simulink model "simulation_basic_working"  (R2022b)
settings: Solver=ode4  StartTime=0.0  StopTime=30  FixedStep=5e-7  MaxStep=1e-6  RelTol=1e-3
undefined symbols (not defined in the file or in its folder): control, inverter, motor, speed
libraries: mcbcontrolslib x5, slpidlib x3, SignalEditorBlockLib x2, spsTriangleGeneratorLib x1
settings Model: Creator=Rizwan Sadik  LastModifiedBy=Rizwan Sadik

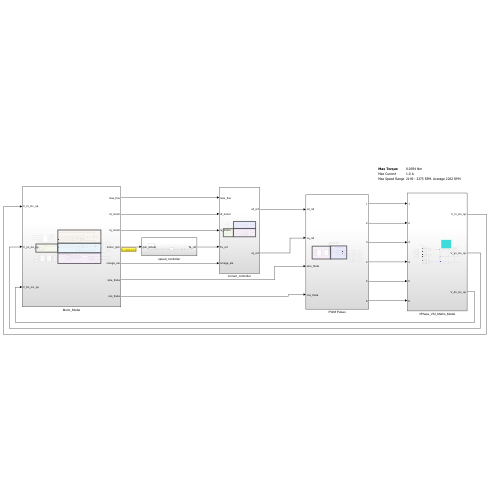
[thumbnail: Simulink's stored preview of the top-level diagram]
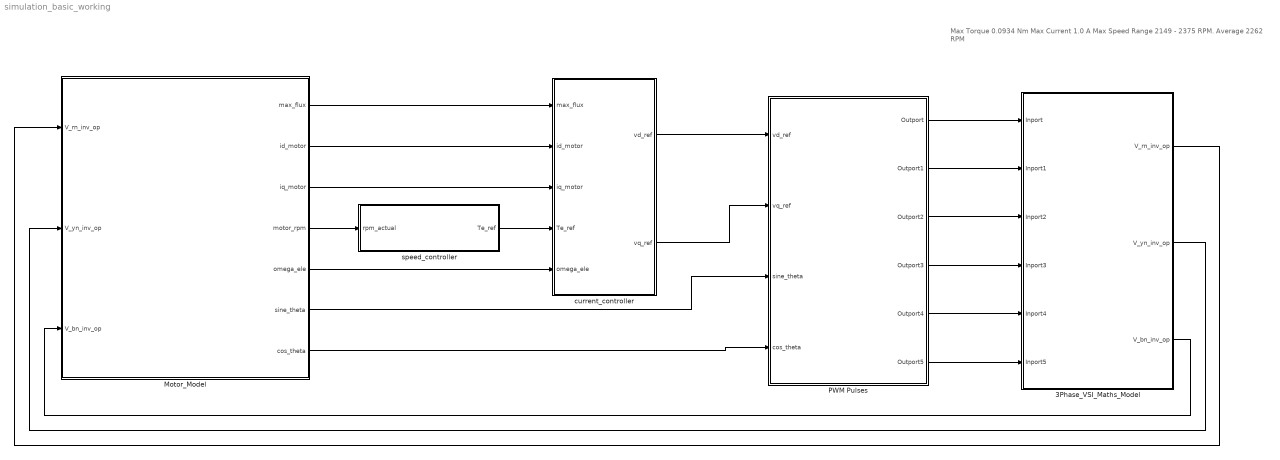
== system simulation_basic_working ==
  note: Max Torque
      | 0.0934 Nm
      |
      | Max Current
      | 1.0 A
      |
      | Max Speed Range
      | 2149 - 2375 RPM. Average 2262 RPM
  3Phase_VSI_Maths_Model : Subsystem  Description=|
      | Input DC Voltage = Vdc
      | Ouput Phase Voltages = Vrn, Vyn, Vbn
      | 
      | Pole Voltage = Vdc/2
      | Pole Voltages - instantaneous values:
      | Vro = +- Vdc/2
      | Vyo = +- Vdc/2
      | Vbo = +- Vdc/2
      | 
      | Leg 1 o/p is Vr. Switches 1 & 4
      | sw 1 ON (sw 4 OFF) -> Vro = +Vdc/2
      | sw 4 ON (sw 1 OFF) -> Vro = -Vdc/2
      | 
      | Leg 2 o/p is Vy. Switches 3 & 6
      | sw 3 ON (sw 6 OFF) -> Vyo = +Vdc/2
      | sw 6 ON (sw 3 OFF) -> Vyo = -Vdc/2
      | 
      | Leg 3 o/p is Vb. Switches 5 & 2
      | sw 5 ON (sw 2 OFF) -> Vbo = +Vdc/2
      | sw 2 ON (sw 5 OFF) -> Vbo = -Vdc/2
      | 
      | Vrn = (2Vro-Vyo-Vbo)/3
      | Vyn = (2Vyo-Vro-Vbo)/3
      | Vbn =(2Vbo-Vyo-Vro)/3
  Motor_Model : Subsystem
  PWM Pulses : Subsystem
  current_controller : Subsystem
  speed_controller : Subsystem
  wires:
  speed_controller/1(Te_ref) -> current_controller/4(Te_ref)
  Motor_Model/5(omega_ele) -> current_controller/5(omega_ele)
  PWM Pulses/1(Outport) -> 3Phase_VSI_Maths_Model/1(Inport)
  Motor_Model/1(max_flux) -> current_controller/1(max_flux)
  PWM Pulses/4(Outport3) -> 3Phase_VSI_Maths_Model/4(Inport3)
  PWM Pulses/5(Outport4) -> 3Phase_VSI_Maths_Model/5(Inport4)
  Motor_Model/6(sine_theta) -> PWM Pulses/3(sine_theta)
  PWM Pulses/3(Outport2) -> 3Phase_VSI_Maths_Model/3(Inport2)
  Motor_Model/3(iq_motor) -> current_controller/3(iq_motor)
  PWM Pulses/2(Outport1) -> 3Phase_VSI_Maths_Model/2(Inport1)
  PWM Pulses/6(Outport5) -> 3Phase_VSI_Maths_Model/6(Inport5)
  Motor_Model/2(id_motor) -> current_controller/2(id_motor)
  Motor_Model/7(cos_theta) -> PWM Pulses/4(cos_theta)
  current_controller/2(vq_ref) -> PWM Pulses/2(vq_ref)
  current_controller/1(vd_ref) -> PWM Pulses/1(vd_ref)
  3Phase_VSI_Maths_Model/3(V_bn_inv_op) -> Motor_Model/3(V_bn_inv_op)
  3Phase_VSI_Maths_Model/2(V_yn_inv_op) -> Motor_Model/2(V_yn_inv_op)
  3Phase_VSI_Maths_Model/1(V_rn_inv_op) -> Motor_Model/1(V_rn_inv_op)
  Motor_Model/4(motor_rpm) -> speed_controller/1(rpm_actual)

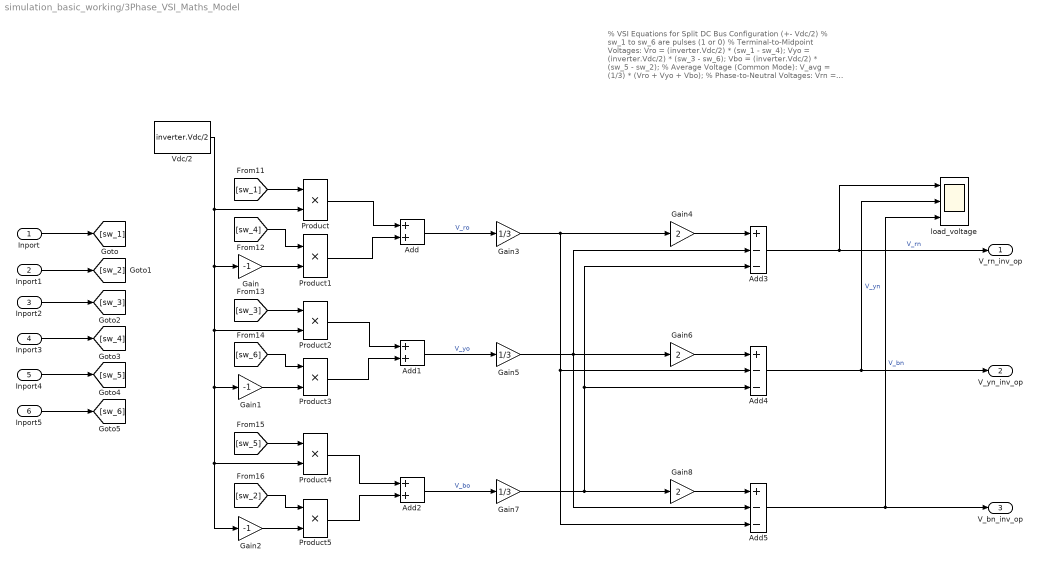
== system simulation_basic_working/3Phase_VSI_Maths_Model ==
  note: % VSI Equations for Split DC Bus Configuration (+- Vdc/2)
      | % sw_1 to sw_6 are pulses (1 or 0)
      |
      | % Terminal-to-Midpoint Voltages:
      | Vro = (inverter.Vdc/2) * (sw_1 - sw_4);
      | Vyo = (inverter.Vdc/2) * (sw_3 - sw_6);
      | Vbo = (inverter.Vdc/2) * (sw_5 - sw_2);
      |
      | % Average Voltage (Common Mode):
      | V_avg = (1/3) * (Vro + Vyo + Vbo);
      |
      | % Phase-to-Neutral Voltages:
      | Vrn = Vro - V_avg;
      | Vyn = Vyo - V_avg;
      | Vbn = Vbo - V_avg;
  Inport : Inport
  Inport1 : Inport  Port=2
  Inport2 : Inport  Port=3
  Inport3 : Inport  Port=4
  Inport4 : Inport  Port=5
  Inport5 : Inport  Port=6
  Add : Sum
  Add1 : Sum
  Add2 : Sum
  Add3 : Sum  Inputs=+--
  Add4 : Sum  Inputs=+--
  Add5 : Sum  Inputs=+--
  Gain : Gain  Gain=-1
  Gain1 : Gain  Gain=-1
  Gain2 : Gain  Gain=-1
  Gain3 : Gain  Gain=1/3
  Gain4 : Gain  Gain=2
  Gain5 : Gain  Gain=1/3
  Gain6 : Gain  Gain=2
  Gain7 : Gain  Gain=1/3
  Gain8 : Gain  Gain=2
  Product{,1..5} (6 alike) : Product
  Vdc/2 : Constant  Value=inverter.Vdc/2
  load_voltage : Scope  NumInputPorts=3
  V_rn_inv_op : Outport
  V_yn_inv_op : Outport  Port=2
  V_bn_inv_op : Outport  Port=3
  wires:
  Product2/1 -> Add1/1
  Add3/1 -> load_voltage/1, V_rn_inv_op/1  "V_rn"
  Product/1 -> Add/1
  Product4/1 -> Add2/1
  Vdc/2/1 -> Gain2/1, Product4/2, Gain1/1, Product2/2, Gain/1, Product/2
  Gain3/1 -> Add5/3, Add4/2, Gain4/1
  Add4/1 -> load_voltage/2, V_yn_inv_op/1  "V_yn"
  [sw_5] -> Product4/1
  Add/1 -> Gain3/1  "V_ro"
  Gain8/1 -> Add5/1
  Add2/1 -> Gain7/1  "V_bo"
  Gain7/1 -> Gain8/1, Add3/3, Add4/3
  Product5/1 -> Add2/2
  Gain5/1 -> Add5/2, Gain6/1, Add3/2
  [sw_3] -> Product2/1
  Gain4/1 -> Add3/1
  [sw_6] -> Product3/1
  Product3/1 -> Add1/2
  [sw_2] -> Product5/1
  Gain1/1 -> Product3/2
  Gain/1 -> Product1/2
  Product1/1 -> Add/2
  [sw_4] -> Product1/1
  [sw_1] -> Product/1
  Gain2/1 -> Product5/2
  Gain6/1 -> Add4/1
  Add5/1 -> V_bn_inv_op/1, load_voltage/3  "V_bn"
  Inport/1 -> [sw_1]
  Inport1/1 -> [sw_2]
  Inport3/1 -> [sw_4]
  Inport2/1 -> [sw_3]
  Inport5/1 -> [sw_6]
  Inport4/1 -> [sw_5]
  Add1/1 -> Gain5/1  "V_yo"

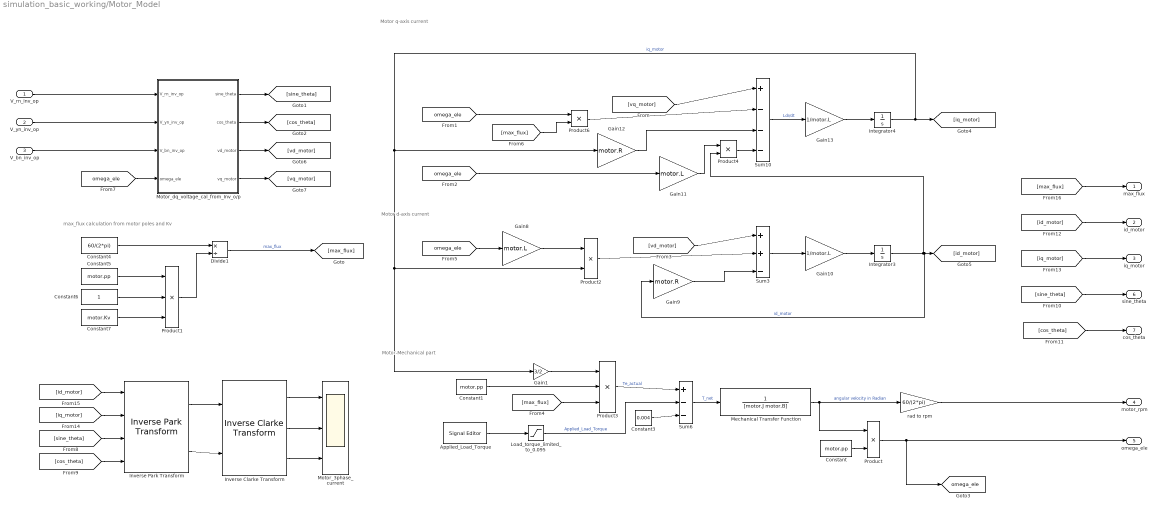
== system simulation_basic_working/Motor_Model ==
  note: max_flux calculation from motor poles and Kv
  note: Motor-Mechanical part
  note: Motor d-axis current
  note: Motor q-axis current
  V_rn_inv_op : Inport
  V_yn_inv_op : Inport  Port=2
  V_bn_inv_op : Inport  Port=3
  Applied_Load_Torque : SignalEditorBlockLib/Signal Editor  FileName=signal_editor.mat  ActiveScenario=Scenario  ActiveSignal=1  IsBus=off  OutputBusObjectStr=Bus: BusObject  SampleTime=0  ZeroCross=off  OutputAfterFinalValue=Setting to zero  Unit=inherit  PreserveSignalName=on
  Constant : Constant  Value=motor.pp
  Constant1 : Constant  Value=motor.pp
  Constant3 : Constant  Value=0.004
  Constant4 : Constant  Value=60/(2*pi)
  Constant5 : Constant  Value=motor.pp
  Constant6 : Constant
  Constant7 : Constant  Value=motor.Kv
  Divide1 : Product  Inputs=*/
  Gain1 : Gain  Gain=3/2
  Gain10 : Gain  Gain=1/motor.L
  Gain11 : Gain  Gain=motor.L
  Gain12 : Gain  Gain=motor.R
  Gain13 : Gain  Gain=1/motor.L
  Gain8 : Gain  Gain=motor.L
  Gain9 : Gain  Gain=motor.R
  Integrator3 : Integrator
  Integrator4 : Integrator
  Inverse Clarke Transform : mcbcontrolslib/Inverse Clarke Transform
      settings: LibrarySourceBlock=mcbhdllib/Controls/Math Transforms/Inverse Clarke Transform
  Inverse Park Transform : mcbcontrolslib/Inverse Park Transform  AxisAlignment=D-axis
      settings: LibrarySourceBlock=mcblib/Controls/Math Transforms/Inverse Park Transform
  Load_torque_limited_to_0.095 : Saturate  UpperLimit=0.095  LowerLimit=0
  Mechanical Transfer Function : TransferFcn  Denominator=[motor.J motor.B]
  Motor_3phase_current : Scope  NumInputPorts=3
  Motor_dq_voltage_cal_from_Inv_o/p : Subsystem
  Product{,2,4,6} (4 alike) : Product
  Product1 : Product  Inputs=3
  Product3 : Product  Inputs=3
  Sum10 : Sum  Inputs=|+---
  Sum3 : Sum  Inputs=|++-
  Sum6 : Sum  Inputs=+|--
  rad to rpm : Gain  Gain=60/(2*pi)
  max_flux : Outport
  id_motor : Outport  Port=2
  iq_motor : Outport  Port=3
  motor_rpm : Outport  Port=4
  omega_ele : Outport  Port=5
  sine_theta : Outport  Port=6
  cos_theta : Outport  Port=7
  tag scope: omega_ele=global
  wires:
  Product6/1 -> Sum10/2
  Gain12/1 -> Sum10/3
  [max_flux] -> Product6/2
  Gain13/1 -> Integrator4/1
  Gain11/1 -> Product4/1
  Integrator4/1 -> [iq_motor], Gain1/1, Product2/2, Gain12/1  "iq_motor"
  Product4/1 -> Sum10/4
  [omega_ele] -> Gain11/1
  Sum10/1 -> Gain13/1  "Ldi/dt​​"
  [vq_motor] -> Sum10/1
  [omega_ele] -> Product6/1
  Product2/1 -> Sum3/2
  Integrator3/1 -> [id_motor], Gain9/1, Product4/2  "id_motor"
  Gain9/1 -> Sum3/3
  Gain8/1 -> Product2/1
  Sum3/1 -> Gain10/1
  Gain10/1 -> Integrator3/1
  [omega_ele] -> Gain8/1
  [vd_motor] -> Sum3/1
  [max_flux] -> Product3/3
  Constant/1 -> Product/2
  Product/1 -> omega_ele/1, [omega_ele]
  Mechanical Transfer Function/1 -> rad to rpm/1, Product/1  "angular velocity in Radian"
  Sum6/1 -> Mechanical Transfer Function/1  "T_net"
  Constant3/1 -> Sum6/3
  Gain1/1 -> Product3/1
  Product3/1 -> Sum6/1  "Te_actual"
  Load_torque_limited_to_0.095/1 -> Sum6/2  "Applied_Load_Torque"
  Constant1/1 -> Product3/2
  rad to rpm/1 -> motor_rpm/1
  Constant6/1 -> Product1/2
  Product1/1 -> Divide1/2
  Constant5/1 -> Product1/1
  Constant7/1 -> Product1/3
  Constant4/1 -> Divide1/1
  Divide1/1 -> [max_flux]  "max_flux"
  Applied_Load_Torque/1 -> Load_torque_limited_to_0.095/1
  V_rn_inv_op/1 -> Motor_dq_voltage_cal_from_Inv_o/p/1(V_rn_inv_op)
  V_yn_inv_op/1 -> Motor_dq_voltage_cal_from_Inv_o/p/2(V_yn_inv_op)
  V_bn_inv_op/1 -> Motor_dq_voltage_cal_from_Inv_o/p/3(V_bn_inv_op)
  [omega_ele] -> Motor_dq_voltage_cal_from_Inv_o/p/4(omega_ele)
  Motor_dq_voltage_cal_from_Inv_o/p/2(cos_theta) -> [cos_theta]
  Motor_dq_voltage_cal_from_Inv_o/p/3(vd_motor) -> [vd_motor]
  Motor_dq_voltage_cal_from_Inv_o/p/4(vq_motor) -> [vq_motor]
  Inverse Clarke Transform/2 -> Motor_3phase_current/2
  Inverse Clarke Transform/1 -> Motor_3phase_current/1
  Inverse Park Transform/1 -> Inverse Clarke Transform/1
  Inverse Clarke Transform/3 -> Motor_3phase_current/3
  Inverse Park Transform/2 -> Inverse Clarke Transform/2
  Motor_dq_voltage_cal_from_Inv_o/p/1(sine_theta) -> [sine_theta]
  [sine_theta] -> Inverse Park Transform/3
  [cos_theta] -> Inverse Park Transform/4
  [sine_theta] -> sine_theta/1
  [cos_theta] -> cos_theta/1
  [id_motor] -> id_motor/1
  [iq_motor] -> iq_motor/1
  [iq_motor] -> Inverse Park Transform/2
  [id_motor] -> Inverse Park Transform/1
  [max_flux] -> max_flux/1

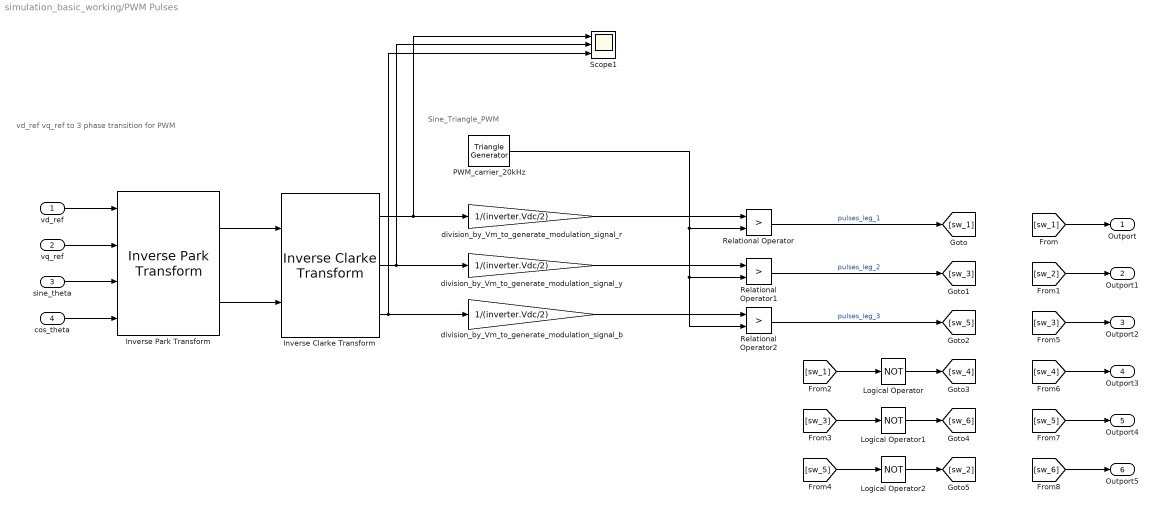
== system simulation_basic_working/PWM Pulses ==
  note: vd_ref vq_ref to 3 phase transition for PWM
  note: Sine_Triangle_PWM
  vd_ref : Inport
  vq_ref : Inport  Port=2
  sine_theta : Inport  Port=3
  cos_theta : Inport  Port=4
  Inverse Clarke Transform : mcbcontrolslib/Inverse Clarke Transform
      settings: LibrarySourceBlock=mcbhdllib/Controls/Math Transforms/Inverse Clarke Transform
  Inverse Park Transform : mcbcontrolslib/Inverse Park Transform  AxisAlignment=D-axis
      settings: LibrarySourceBlock=mcblib/Controls/Math Transforms/Inverse Park Transform
  Logical Operator : Logic  Operator=NOT  AllPortsSameDT=off  OutDataTypeStr=boolean
  Logical Operator1 : Logic  Operator=NOT  AllPortsSameDT=off  OutDataTypeStr=boolean
  Logical Operator2 : Logic  Operator=NOT  AllPortsSameDT=off  OutDataTypeStr=boolean
  PWM_carrier_20kHz : spsTriangleGeneratorLib/Triangle Generator  Freq=20000  Phase=0  Ts=0
  Relational Operator : RelationalOperator  Operator=>  OutDataTypeStr=boolean  RndMeth=Simplest  InputSameDT=off
  Relational Operator1 : RelationalOperator  Operator=>  OutDataTypeStr=boolean  RndMeth=Simplest  InputSameDT=off
  Relational Operator2 : RelationalOperator  Operator=>  OutDataTypeStr=boolean  RndMeth=Simplest  InputSameDT=off
  Scope1 : Scope  NumInputPorts=3
  division_by_Vm_to_generate_modulation_signal_b : Gain  Gain=1/(inverter.Vdc/2)
  division_by_Vm_to_generate_modulation_signal_r : Gain  Gain=1/(inverter.Vdc/2)
  division_by_Vm_to_generate_modulation_signal_y : Gain  Gain=1/(inverter.Vdc/2)
  Outport : Outport
  Outport1 : Outport  Port=2
  Outport2 : Outport  Port=3
  Outport3 : Outport  Port=4
  Outport4 : Outport  Port=5
  Outport5 : Outport  Port=6
  wires:
  [sw_3] -> Logical Operator1/1
  Logical Operator2/1 -> [sw_2]
  cos_theta/1 -> Inverse Park Transform/4
  sine_theta/1 -> Inverse Park Transform/3
  [sw_5] -> Logical Operator2/1
  Inverse Park Transform/2 -> Inverse Clarke Transform/2
  Inverse Park Transform/1 -> Inverse Clarke Transform/1
  Logical Operator/1 -> [sw_4]
  Logical Operator1/1 -> [sw_6]
  [sw_1] -> Logical Operator/1
  vd_ref/1 -> Inverse Park Transform/1
  vq_ref/1 -> Inverse Park Transform/2
  [sw_1] -> Outport/1
  [sw_6] -> Outport5/1
  [sw_2] -> Outport1/1
  [sw_3] -> Outport2/1
  [sw_4] -> Outport3/1
  [sw_5] -> Outport4/1
  Relational Operator2/1 -> [sw_5]  "pulses_leg_3"
  Relational Operator1/1 -> [sw_3]  "pulses_leg_2"
  Relational Operator/1 -> [sw_1]  "pulses_leg_1"
  PWM_carrier_20kHz/1 -> Relational Operator2/2, Relational Operator1/2, Relational Operator/2
  division_by_Vm_to_generate_modulation_signal_y/1 -> Relational Operator1/1
  division_by_Vm_to_generate_modulation_signal_b/1 -> Relational Operator2/1
  Inverse Clarke Transform/3 -> Scope1/3, division_by_Vm_to_generate_modulation_signal_b/1
  Inverse Clarke Transform/2 -> Scope1/2, division_by_Vm_to_generate_modulation_signal_y/1
  division_by_Vm_to_generate_modulation_signal_r/1 -> Relational Operator/1
  Inverse Clarke Transform/1 -> Scope1/1, division_by_Vm_to_generate_modulation_signal_r/1

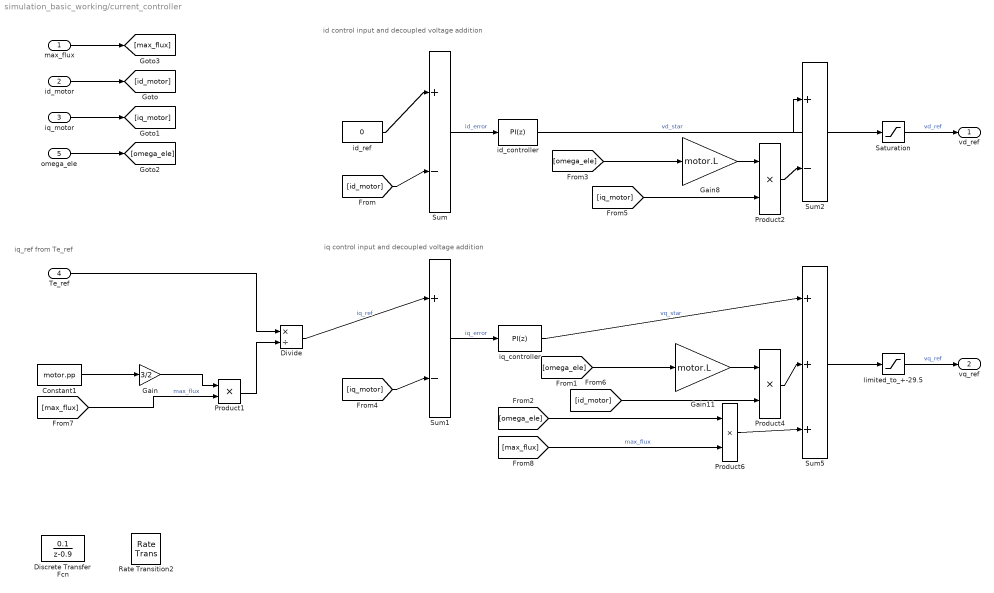
== system simulation_basic_working/current_controller ==
  note: iq_ref from Te_ref
  note: iq control input and decoupled voltage addition
  note: id control input and decoupled voltage addition
  max_flux : Inport
  id_motor : Inport  Port=2
  iq_motor : Inport  Port=3
  Te_ref : Inport  Port=4  SampleTime=5e-4
  omega_ele : Inport  Port=5
  Constant1 : Constant  Value=motor.pp
  Discrete Transfer Fcn : DiscreteTransferFcn  Numerator=[0.1]  Denominator=[1 -0.9]  SampleTime=5e-5
  Divide : Product  Inputs=*/
  Gain : Gain  Gain=3/2
  Gain11 : Gain  Gain=motor.L
  Gain8 : Gain  Gain=motor.L
  Product{1..2,4,6} (4 alike) : Product
  Rate Transition2 : RateTransition  Integrity=off  OutPortSampleTime=5e-5
  Saturation : Saturate  UpperLimit=29.5  LowerLimit=-29.5
  Sum : Sum  Inputs=|+-
  Sum1 : Sum  Inputs=|+-
  Sum2 : Sum  Inputs=|+-
  Sum5 : Sum  Inputs=|+++
  id_controller : slpidlib/PID Controller  Controller=PI  Form=Parallel  TimeDomain=Discrete-time  UseExternalTs=off  SampleTime=5e-5  IntegratorMethod=Forward Euler  FilterMethod=Forward Euler  ControllerParametersSource=internal  P=control.Kp  I=control.Ki  UseKiTs=off  D=0  N=100  UseFilter=on  TunerSelectOption=Transfer Function Based (PID Tuner App)  InitialConditionSource=internal  InitialConditionForIntegrator=0  InitialConditionForFilter=0  DifferentiatorICPrevScaledInput=0  ExternalReset=none  TrackingMode=off  Kt=1  LimitOutput=on  SatLimitsSource=internal  UpperSaturationLimit=inf  LowerSaturationLimit=-inf  LinearizeAsGain=on  AntiWindupMode=clamping  Kb=1  LimitIntegrator=off  UpperIntegratorSaturationLimit=inf  LowerIntegratorSaturationLimit=-inf  POutMin=[]  POutMax=[]  IOutMin=[]  IOutMax=[]  DOutMin=[]  DOutMax=[]  NOutMin=[]  NOutMax=[]  SumOutMin=[]  SumOutMax=[]  SaturationOutMin=[]  SaturationOutMax=[]  PParamMin=[]  PParamMax=[]  IParamMin=[]  IParamMax=[]  DParamMin=[]  DParamMax=[]  NParamMin=[]  NParamMax=[]  KbParamMin=[]  KbParamMax=[]  KtParamMin=[]  KtParamMax=[]  KbOutMin=[]  KbOutMax=[]  KtOutMin=[]  KtOutMax=[]  IntegratorOutMin=[]  IntegratorOutMax=[]  FilterOutMin=[]  FilterOutMax=[]  SumI1OutMin=[]  SumI1OutMax=[]  SumI2OutMin=[]  SumI2OutMax=[]  SumI3OutMin=[]  SumI3OutMax=[]  SumI4OutMin=[]  SumI4OutMax=[]  SumDOutMin=[]  SumDOutMax=[]  DifferentiatorOutMin=[]  DifferentiatorOutMax=[]  FilterDiffOutCoefMin=[]  FilterDiffOutCoefMax=[]  ReciprocalOutMin=[]  ReciprocalOutMax=[]  SumDenOutMin=[]  SumDenOutMax=[]  SumNumOutMin=[]  SumNumOutMax=[]  DivideOutMin=[]  DivideOutMax=[]  UdiffTsProdOutMin=[]  UdiffTsProdOutMax=[]  NTsProdOutMin=[]  NTsProdOutMax=[]  UintegralTsProdOutMin=[]  UintegralTsProdOutMax=[]  UngainTsProdOutMin=[]  UngainTsProdOutMax=[]  ClampingZeroOutDataTypeStr=Inherit: Inherit via back propagation  ClampingZeroOutMin=[]  ClampingZeroOutMax=[]  FilterDenConstantOutDataTypeStr=Inherit: Inherit via back propagation  FilterDenConstantOutMin=[]  FilterDenConstantOutMax=[]  PCopyOutDataTypeStr=Inherit: Inherit via back propagation  PCopyOutMin=[]  PCopyOutMax=[]  NCopyOutDataTypeStr=Inherit: Inherit via back propagation  NCopyOutMin=[]  NCopyOutMax=[]  IntegratorContinuousStateAttributes=''  IntegratorStateMustResolveToSignalObject=off  IntegratorRTWStateStorageClass=Auto  FilterContinuousStateAttributes=''  FilterStateMustResolveToSignalObject=off  FilterRTWStateStorageClass=Auto  ParallelPVariant=InternalParameters  IdealPVariant=Disabled  IVariant=InternalParameters  DVariant=Disabled  IntegratorVariant=Discrete  SatVariant=Enabled  AWVariant=DiscClampingParallel  PCopyVariant=Disabled  TRVariant=Disabled  FdbkBlocksVariant=Forward  IdealPFdbkVariant=Disabled  SatFdbkVariant=Disabled  DerivativeFilterVariant=Disabled  NVariant=Disabled  NCopyVariant=Disabled_SignalSpec  FilterICVariant=Disabled  IntegratorICVariant=InternalICs  ExternalResetVariant=Disabled  TRSumVariant=Passthrough  SumFdbkVariant=Disabled  SumVariant=Sum_PI  TsampFilterVariant=InternalTs  TsampNgainVariant=Passthrough  TsampIntegralVariant=Passthrough  ExternalSaturationOutDataTypeStr=Inherit: Same as second input
  id_ref : Constant  Value=0
  iq_controller : slpidlib/PID Controller  Controller=PI  Form=Parallel  TimeDomain=Discrete-time  UseExternalTs=off  SampleTime=5e-5  IntegratorMethod=Forward Euler  FilterMethod=Forward Euler  ControllerParametersSource=internal  P=control.Kp*1  I=control.Ki  UseKiTs=off  D=0  N=100  UseFilter=on  TunerSelectOption=Transfer Function Based (PID Tuner App)  InitialConditionSource=internal  InitialConditionForIntegrator=0  InitialConditionForFilter=0  DifferentiatorICPrevScaledInput=0  ExternalReset=none  TrackingMode=off  Kt=1  LimitOutput=on  SatLimitsSource=internal  UpperSaturationLimit=inf  LowerSaturationLimit=-inf  LinearizeAsGain=on  AntiWindupMode=clamping  Kb=1  LimitIntegrator=on  UpperIntegratorSaturationLimit=29.5  LowerIntegratorSaturationLimit=-29.5  POutMin=[]  POutMax=[]  IOutMin=[]  IOutMax=[]  DOutMin=[]  DOutMax=[]  NOutMin=[]  NOutMax=[]  SumOutMin=[]  SumOutMax=[]  SaturationOutMin=[]  SaturationOutMax=[]  PParamMin=[]  PParamMax=[]  IParamMin=[]  IParamMax=[]  DParamMin=[]  DParamMax=[]  NParamMin=[]  NParamMax=[]  KbParamMin=[]  KbParamMax=[]  KtParamMin=[]  KtParamMax=[]  KbOutMin=[]  KbOutMax=[]  KtOutMin=[]  KtOutMax=[]  IntegratorOutMin=[]  IntegratorOutMax=[]  FilterOutMin=[]  FilterOutMax=[]  SumI1OutMin=[]  SumI1OutMax=[]  SumI2OutMin=[]  SumI2OutMax=[]  SumI3OutMin=[]  SumI3OutMax=[]  SumI4OutMin=[]  SumI4OutMax=[]  SumDOutMin=[]  SumDOutMax=[]  DifferentiatorOutMin=[]  DifferentiatorOutMax=[]  FilterDiffOutCoefMin=[]  FilterDiffOutCoefMax=[]  ReciprocalOutMin=[]  ReciprocalOutMax=[]  SumDenOutMin=[]  SumDenOutMax=[]  SumNumOutMin=[]  SumNumOutMax=[]  DivideOutMin=[]  DivideOutMax=[]  UdiffTsProdOutMin=[]  UdiffTsProdOutMax=[]  NTsProdOutMin=[]  NTsProdOutMax=[]  UintegralTsProdOutMin=[]  UintegralTsProdOutMax=[]  UngainTsProdOutMin=[]  UngainTsProdOutMax=[]  ClampingZeroOutDataTypeStr=Inherit: Inherit via back propagation  ClampingZeroOutMin=[]  ClampingZeroOutMax=[]  FilterDenConstantOutDataTypeStr=Inherit: Inherit via back propagation  FilterDenConstantOutMin=[]  FilterDenConstantOutMax=[]  PCopyOutDataTypeStr=Inherit: Inherit via back propagation  PCopyOutMin=[]  PCopyOutMax=[]  NCopyOutDataTypeStr=Inherit: Inherit via back propagation  NCopyOutMin=[]  NCopyOutMax=[]  IntegratorContinuousStateAttributes=''  IntegratorStateMustResolveToSignalObject=off  IntegratorRTWStateStorageClass=Auto  FilterContinuousStateAttributes=''  FilterStateMustResolveToSignalObject=off  FilterRTWStateStorageClass=Auto  ParallelPVariant=InternalParameters  IdealPVariant=Disabled  IVariant=InternalParameters  DVariant=Disabled  IntegratorVariant=Discrete  SatVariant=Enabled  AWVariant=DiscClampingParallel  PCopyVariant=Disabled  TRVariant=Disabled  FdbkBlocksVariant=Forward  IdealPFdbkVariant=Disabled  SatFdbkVariant=Disabled  DerivativeFilterVariant=Disabled  NVariant=Disabled  NCopyVariant=Disabled_SignalSpec  FilterICVariant=Disabled  IntegratorICVariant=InternalICs  ExternalResetVariant=Disabled  TRSumVariant=Passthrough  SumFdbkVariant=Disabled  SumVariant=Sum_PI  TsampFilterVariant=InternalTs  TsampNgainVariant=Passthrough  TsampIntegralVariant=Passthrough  ExternalSaturationOutDataTypeStr=Inherit: Same as second input
  limited_to_+-29.5 : Saturate  UpperLimit=29.5  LowerLimit=-29.5
  vd_ref : Outport
  vq_ref : Outport  Port=2
  wires:
  Sum1/1 -> iq_controller/1  "iq_error"
  id_motor/1 -> [id_motor]
  Te_ref/1 -> Divide/1
  Sum5/1 -> limited_to_+-29.5/1
  limited_to_+-29.5/1 -> vq_ref/1  "vq_ref"
  Product4/1 -> Sum5/2
  Product6/1 -> Sum5/3
  iq_controller/1 -> Sum5/1  "vq_star"
  max_flux/1 -> [max_flux]
  Product2/1 -> Sum2/2
  Gain8/1 -> Product2/1
  Sum2/1 -> Saturation/1
  iq_motor/1 -> [iq_motor]
  id_controller/1 -> Sum2/1  "vd_star"
  id_ref/1 -> Sum/1
  Sum/1 -> id_controller/1  "id_error"
  Saturation/1 -> vd_ref/1  "vd_ref"
  [id_motor] -> Sum/2
  omega_ele/1 -> [omega_ele]
  [omega_ele] -> Product6/1
  [iq_motor] -> Sum1/2
  Gain11/1 -> Product4/1
  Product1/1 -> Divide/2
  Gain/1 -> Product1/1
  Constant1/1 -> Gain/1
  [max_flux] -> Product1/2  "max_flux"
  [max_flux] -> Product6/2  "max_flux"
  Divide/1 -> Sum1/1  "iq_ref"
  [omega_ele] -> Gain8/1
  [iq_motor] -> Product2/2
  [id_motor] -> Product4/2
  [omega_ele] -> Gain11/1

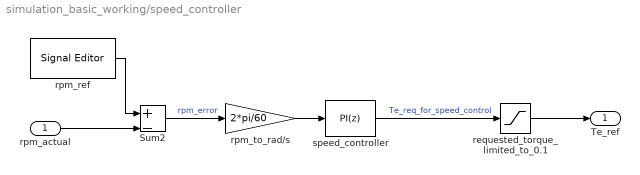
== system simulation_basic_working/speed_controller ==
  rpm_actual : Inport
  Sum2 : Sum  Inputs=|+-
  requested_torque_limited_to_0.1 : Saturate  UpperLimit=0.1  LowerLimit=-0.05
  rpm_ref : SignalEditorBlockLib/Signal Editor  FileName=signal_editor.mat  ActiveScenario=Scenario1  ActiveSignal=Signal  IsBus=off  OutputBusObjectStr=Bus: BusObject  SampleTime=0  ZeroCross=off  OutputAfterFinalValue=Setting to zero  Unit=inherit  PreserveSignalName=on
  rpm_to_rad/s : Gain  Gain=2*pi/60
  speed_controller : slpidlib/PID Controller  Controller=PI  Form=Parallel  TimeDomain=Discrete-time  UseExternalTs=off  SampleTime=1/2000  IntegratorMethod=Forward Euler  FilterMethod=Forward Euler  ControllerParametersSource=internal  P=speed.ke  I=speed.ki  UseKiTs=off  D=0  N=100  UseFilter=on  TunerSelectOption=Transfer Function Based (PID Tuner App)  InitialConditionSource=internal  InitialConditionForIntegrator=0  InitialConditionForFilter=0  DifferentiatorICPrevScaledInput=0  ExternalReset=none  TrackingMode=off  Kt=1  LimitOutput=on  SatLimitsSource=internal  UpperSaturationLimit=0.1  LowerSaturationLimit=-0.05  LinearizeAsGain=off  AntiWindupMode=clamping  Kb=1  LimitIntegrator=on  UpperIntegratorSaturationLimit=0.1  LowerIntegratorSaturationLimit=0  POutMin=[]  POutMax=[]  IOutMin=[]  IOutMax=[]  DOutMin=[]  DOutMax=[]  NOutMin=[]  NOutMax=[]  SumOutMin=[]  SumOutMax=[]  SaturationOutMin=[]  SaturationOutMax=[]  PParamMin=[]  PParamMax=[]  IParamMin=[]  IParamMax=[]  DParamMin=[]  DParamMax=[]  NParamMin=[]  NParamMax=[]  KbParamMin=[]  KbParamMax=[]  KtParamMin=[]  KtParamMax=[]  KbOutMin=[]  KbOutMax=[]  KtOutMin=[]  KtOutMax=[]  IntegratorOutMin=[]  IntegratorOutMax=[]  FilterOutMin=[]  FilterOutMax=[]  SumI1OutMin=[]  SumI1OutMax=[]  SumI2OutMin=[]  SumI2OutMax=[]  SumI3OutMin=[]  SumI3OutMax=[]  SumI4OutMin=[]  SumI4OutMax=[]  SumDOutMin=[]  SumDOutMax=[]  DifferentiatorOutMin=[]  DifferentiatorOutMax=[]  FilterDiffOutCoefMin=[]  FilterDiffOutCoefMax=[]  ReciprocalOutMin=[]  ReciprocalOutMax=[]  SumDenOutMin=[]  SumDenOutMax=[]  SumNumOutMin=[]  SumNumOutMax=[]  DivideOutMin=[]  DivideOutMax=[]  UdiffTsProdOutMin=[]  UdiffTsProdOutMax=[]  NTsProdOutMin=[]  NTsProdOutMax=[]  UintegralTsProdOutMin=[]  UintegralTsProdOutMax=[]  UngainTsProdOutMin=[]  UngainTsProdOutMax=[]  ClampingZeroOutDataTypeStr=Inherit: Inherit via back propagation  ClampingZeroOutMin=[]  ClampingZeroOutMax=[]  FilterDenConstantOutDataTypeStr=Inherit: Inherit via back propagation  FilterDenConstantOutMin=[]  FilterDenConstantOutMax=[]  PCopyOutDataTypeStr=Inherit: Inherit via back propagation  PCopyOutMin=[]  PCopyOutMax=[]  NCopyOutDataTypeStr=Inherit: Inherit via back propagation  NCopyOutMin=[]  NCopyOutMax=[]  IntegratorContinuousStateAttributes=''  IntegratorStateMustResolveToSignalObject=off  IntegratorRTWStateStorageClass=Auto  FilterContinuousStateAttributes=''  FilterStateMustResolveToSignalObject=off  FilterRTWStateStorageClass=Auto  ParallelPVariant=InternalParameters  IdealPVariant=Disabled  IVariant=InternalParameters  DVariant=Disabled  IntegratorVariant=Discrete  SatVariant=Enabled  AWVariant=DiscClampingParallel  PCopyVariant=Disabled  TRVariant=Disabled  FdbkBlocksVariant=Forward  IdealPFdbkVariant=Disabled  SatFdbkVariant=Disabled  DerivativeFilterVariant=Disabled  NVariant=Disabled  NCopyVariant=Disabled_SignalSpec  FilterICVariant=Disabled  IntegratorICVariant=InternalICs  ExternalResetVariant=Disabled  TRSumVariant=Passthrough  SumFdbkVariant=Disabled  SumVariant=Sum_PI  TsampFilterVariant=InternalTs  TsampNgainVariant=Passthrough  TsampIntegralVariant=Passthrough  ExternalSaturationOutDataTypeStr=Inherit: Same as second input
  Te_ref : Outport  SampleTime=5e-4
  wires:
  rpm_actual/1 -> Sum2/2
  Sum2/1 -> rpm_to_rad/s/1  "rpm_error"
  speed_controller/1 -> requested_torque_limited_to_0.1/1  "Te_req_for_speed_control"
  requested_torque_limited_to_0.1/1 -> Te_ref/1
  rpm_to_rad/s/1 -> speed_controller/1
  rpm_ref/1 -> Sum2/1

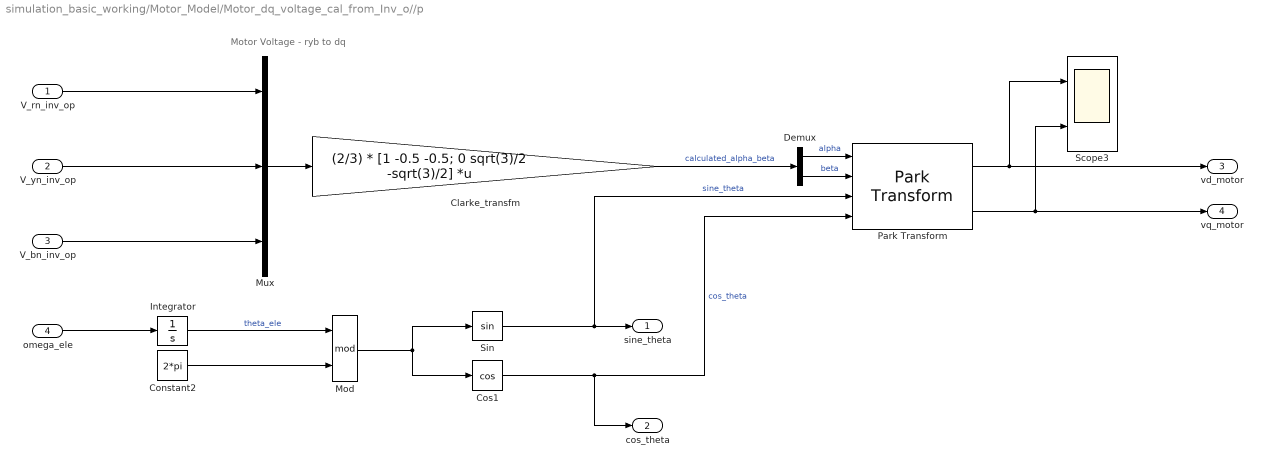
== system simulation_basic_working/Motor_Model/Motor_dq_voltage_cal_from_Inv_o//p ==
  note: Motor Voltage - ryb to dq
  V_rn_inv_op : Inport
  V_yn_inv_op : Inport  Port=2
  V_bn_inv_op : Inport  Port=3
  omega_ele : Inport  Port=4
  Clarke_transfm : Gain  Gain=(2/3) * [1 -0.5 -0.5; 0 sqrt(3)/2 -sqrt(3)/2]  Multiplication=Matrix(K*u)
  Constant2 : Constant  Value=2*pi
  Cos1 : Trigonometry  Operator=cos
  Demux : Demux  Outputs=2
  Integrator : Integrator
  Mod : Math  Operator=mod
  Mux : Mux  Inputs=3
  Park Transform : mcbcontrolslib/Park Transform  AxisAlignment=D-axis
      settings: LibrarySourceBlock=mcbhdllib/Controls/Math Transforms/Park Transform
  Scope3 : Scope  NumInputPorts=2
  Sin : Trigonometry
  sine_theta : Outport
  cos_theta : Outport  Port=2
  vd_motor : Outport  Port=3
  vq_motor : Outport  Port=4
  wires:
  Sin/1 -> sine_theta/1, Park Transform/3  "sine_theta"
  Constant2/1 -> Mod/2
  Cos1/1 -> cos_theta/1, Park Transform/4  "cos_theta"
  Mod/1 -> Cos1/1, Sin/1
  Demux/1 -> Park Transform/1  "alpha"
  Park Transform/2 -> Scope3/2, vq_motor/1
  Clarke_transfm/1 -> Demux/1  "calculated_alpha_beta"
  Integrator/1 -> Mod/1  "theta_ele"
  Demux/2 -> Park Transform/2  "beta"
  Mux/1 -> Clarke_transfm/1
  Park Transform/1 -> vd_motor/1, Scope3/1
  V_bn_inv_op/1 -> Mux/3
  omega_ele/1 -> Integrator/1
  V_rn_inv_op/1 -> Mux/1
  V_yn_inv_op/1 -> Mux/2
